simulink model "controller"  (R2024b)
settings: Solver=FixedStepAuto  StartTime=0.0  StopTime=100  FixedStep=1/100  RelTol=1e-3
undefined symbols (not defined in the file or in its folder): MAX_RDB_ENGAGE_SPEED, MAX_TORQUE, MAX_TORQUE_REVERSE, TransmissionState
settings Model: Creator=DAUIN-Win10  LastModifiedBy=aayan
settings SolverCC: AutoInsertRateTranBlk=on
settings OptimizationCC: ReuseModelBlockBuffer=off
settings DebuggingCC: UnconnectedInputMsg=warning  UnconnectedOutputMsg=warning  UnconnectedLineMsg=warning
settings ModelReferenceCC: EnableRefExpFcnMdlSchedulingChecks=on
settings RTWCC: GPUComputeCapability=3.5  DLArmComputeVersion=19.05

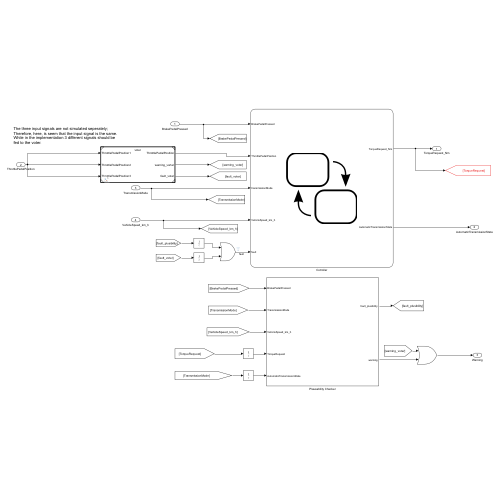
[thumbnail: Simulink's stored preview of the top-level diagram]
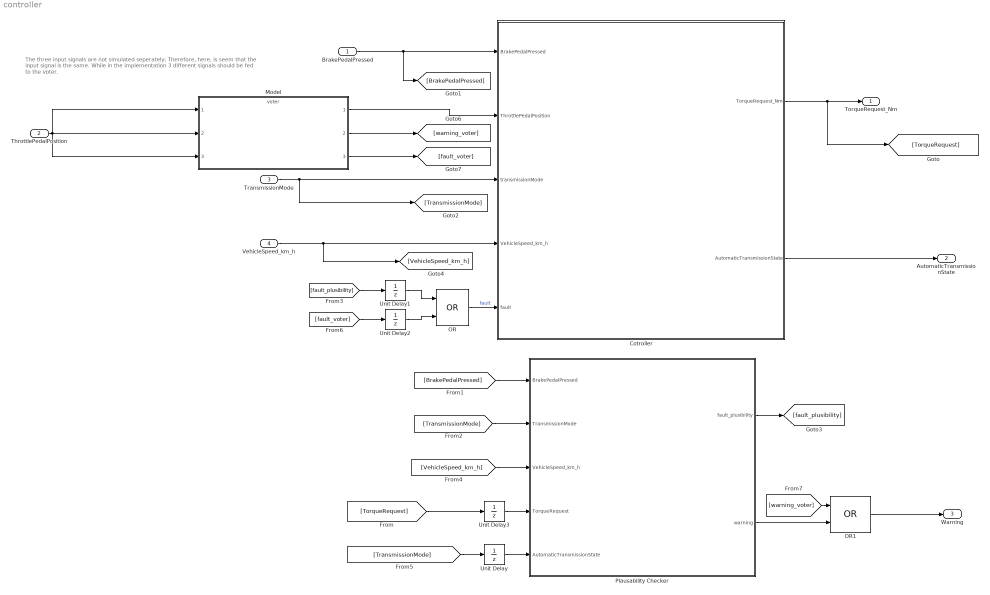
== system controller ==
  note: The three input signals are not simulated seperately;
      | Therefore, here, is seem that the input signal is the same.
      | While in the implementation 3 different signals should be
      | fed to the voter.
  BrakePedalPressed : Inport  OutDataTypeStr=boolean
  ThrottlePedalPosition : Inport  Port=2  OutDataTypeStr=single
  TransmissionMode : Inport  Port=3  OutDataTypeStr=Enum: TransmissionState
  VehicleSpeed_km_h : Inport  Port=4  OutDataTypeStr=single  Unit=km/h
  Cotroller : Stateflow chart  TreatAsAtomicUnit=on
      settings: PortSchema="{\"entries\":[{\"content\":{\"sides\":[{\"content\":{\"connectorIds\":[\"In1\",\"In2\",\"In3\",\"In4\",\"In5\"]},\"type\":\"ConnectorPlacement.EquallySpacedRectSide\",\"uuid\":\"fa3865f3-071a-4523-b56b-dfcb7b7ff1e1\"},{\"content\":{\"connectorIds\":[\"Out2\",\"Out1\"],\"side\":\"RIGHT\"},\"type\":\"ConnectorPlacement.EquallySpacedRectSide\",\"uuid\":\"97edfdd5-6ca1-4319-83ef-4a85a5b2efa4\"},{\"content\":{\"side\":\"TOP\"},\"type\":\"ConnectorPlacement.EquallySpacedRectSide\",\"uuid\":\"bfa350c0-61e1-4051-a5a1-0c01bc7888ec\"}]},\"type\":\"ConnectorPlacement.EquallySpacedConnector\",\"uuid\":\"0069708a-38e0-4c12-a9eb-137e78633e28\"}],\"packageUris\":[\"http://schema.mathworks.com/mf0/Connector/R2020b\"],\"version\":\"1.0\"}"
  Model : ModelReference  ModelNameDialog=voter.slx  SimulationMode=Normal  ModelReferenceVersion=1.25
  OR : Logic  Operator=OR  IconShape=distinctive  AllPortsSameDT=off  OutDataTypeStr=boolean
  OR1 : Logic  Operator=OR  IconShape=distinctive  AllPortsSameDT=off  OutDataTypeStr=boolean
  Plausability Checker : Subsystem
  Unit Delay : UnitDelay  InitialCondition=TransmissionState.Park  SampleTime=-1  HasFrameUpgradeWarning=on
  Unit Delay1 : UnitDelay  SampleTime=-1  HasFrameUpgradeWarning=on
  Unit Delay2 : UnitDelay  SampleTime=-1  HasFrameUpgradeWarning=on
  Unit Delay3 : UnitDelay  SampleTime=-1  HasFrameUpgradeWarning=on
  TorqueRequest_Nm : Outport  OutDataTypeStr=single  Unit=N*m
  AutomaticTransmissionState : Outport  Port=2  OutDataTypeStr=Enum: TransmissionState
  Warning : Outport  Port=3  OutDataTypeStr=boolean
  wires:
  [BrakePedalPressed] -> Plausability Checker/1(BrakePedalPressed)
  [TransmissionMode] -> Plausability Checker/2(TransmissionMode)
  VehicleSpeed_km_h/1 -> [VehicleSpeed_km_h], Cotroller/4(VehicleSpeed_km_h)
  [TorqueRequest] -> Unit Delay3/1
  Plausability Checker/1(fault_plusibility) -> [fault_plusibility]
  [VehicleSpeed_km_h] -> Plausability Checker/3(VehicleSpeed_km_h)
  [TransmissionMode] -> Unit Delay/1
  ThrottlePedalPosition/1 -> Model/3, Model/1, Model/2
  Model/2 -> [warning_voter]
  Model/3 -> [fault_voter]
  OR/1 -> Cotroller/5(fault)  "fault"
  [fault_plusibility] -> Unit Delay1/1
  [fault_voter] -> Unit Delay2/1
  Plausability Checker/2(warning) -> OR1/2
  OR1/1 -> Warning/1
  [warning_voter] -> OR1/1
  BrakePedalPressed/1 -> [BrakePedalPressed], Cotroller/1(BrakePedalPressed)
  TransmissionMode/1 -> [TransmissionMode], Cotroller/3(transmissionMode)
  Model/1 -> Cotroller/2(ThrottlePedalPosition)
  Unit Delay1/1 -> OR/1
  Unit Delay2/1 -> OR/2
  Cotroller/2(TorqueRequest_Nm) -> [TorqueRequest], TorqueRequest_Nm/1
  Cotroller/1(AutomaticTransmissionState) -> AutomaticTransmissionState/1
  Unit Delay/1 -> Plausability Checker/5(AutomaticTransmissionState)
  Unit Delay3/1 -> Plausability Checker/4(TorqueRequest)

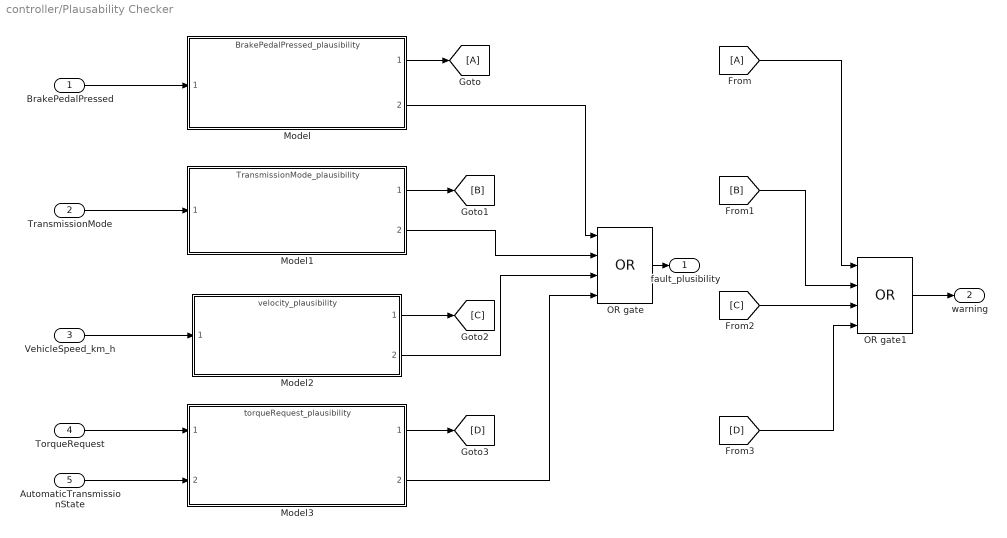
== system controller/Plausability Checker ==
  BrakePedalPressed : Inport
  TransmissionMode : Inport  Port=2  OutDataTypeStr=Enum: TransmissionState
  VehicleSpeed_km_h : Inport  Port=3
  TorqueRequest : Inport  Port=4  OutDataTypeStr=single
  AutomaticTransmissionState : Inport  Port=5  OutDataTypeStr=Enum: TransmissionState
  From : From
  Goto : Goto
  Model : ModelReference  ModelNameDialog=BrakePedalPressed_plausibility.slx  SimulationMode=Normal  ModelReferenceVersion=1.18
  Model1 : ModelReference  ModelNameDialog=TransmissionMode_plausibility.slx  SimulationMode=Normal  ModelReferenceVersion=1.12
  Model2 : ModelReference  ModelNameDialog=velocity_plausibility.slx  SimulationMode=Normal  ModelReferenceVersion=1.13
  Model3 : ModelReference  ModelNameDialog=torqueRequest_plausibility.slx  SimulationMode=Normal  ModelReferenceVersion=1.19
  OR gate : Logic  Operator=OR  Inputs=4  IconShape=distinctive  AllPortsSameDT=off  OutDataTypeStr=boolean
  OR gate1 : Logic  Operator=OR  Inputs=4  IconShape=distinctive  AllPortsSameDT=off  OutDataTypeStr=boolean
  fault_plusibility : Outport  OutDataTypeStr=boolean
  warning : Outport  Port=2
  wires:
  BrakePedalPressed/1 -> Model/1
  Model/1 -> Goto/1
  TransmissionMode/1 -> Model1/1
  Model1/1 -> [B]
  Model/2 -> OR gate/1
  Model1/2 -> OR gate/2
  Model2/2 -> OR gate/3
  AutomaticTransmissionState/1 -> Model3/2
  OR gate1/1 -> warning/1
  Model2/1 -> [C]
  Model3/1 -> [D]
  From/1 -> OR gate1/1
  [B] -> OR gate1/2
  [D] -> OR gate1/4
  [C] -> OR gate1/3
  OR gate/1 -> fault_plusibility/1
  Model3/2 -> OR gate/4
  TorqueRequest/1 -> Model3/1
  VehicleSpeed_km_h/1 -> Model2/1

== stateflow chart controller/Cotroller ==
  settings: updateMethod=DISCRETE  sampleTime=0.01
  state Park
    en:
    AutomaticTransmissionState = TransmissionState.Park;
    du:
    TorqueRequest_Nm = single(0);
  state Neutral
    en:
    AutomaticTransmissionState = TransmissionState.Neutral;
    du:
    TorqueRequest_Nm = single(0);
  state Drive
    en:
    AutomaticTransmissionState = TransmissionState.Drive;
    state ZeroTorque1
      du:
      TorqueRequest_Nm = single(0);
    state Acceleration
      du:
      TorqueRequest_Nm = single(MAX_TORQUE*(ThrottlePedalPosition));
    state StartToMove
      du:
      TorqueRequest_Nm = single(5);
    (default) -> ZeroTorque1
    ZeroTorque1 -> (junction 99) [order 1] : [BrakePedalPressed ~= 1 && VehicleSpeed_km_h  < 5 ]
    (junction 99) -> StartToMove
    (junction 94) -> ZeroTorque1
    StartToMove -> (junction 94) [order 2] : [BrakePedalPressed == 1]
    ZeroTorque1 -> Acceleration [order 2] : [(BrakePedalPressed ~= 1)]
    Acceleration -> ZeroTorque1 : [ (BrakePedalPressed == 1)]
    StartToMove -> Acceleration [order 1] : [ThrottlePedalPosition > 0 && BrakePedalPressed ~= 1]
  state Brake
    en:
    AutomaticTransmissionState = TransmissionState.Brake
    state AccelerationRegion
      du:
      TorqueRequest_Nm = single(MAX_TORQUE*(3/2)*(ThrottlePedalPosition - (1/3)));
    state ZeroTorque
      TorqueRequest_Nm = single(0);
    state DecelerationRegion
      du:
      TorqueRequest_Nm = single(-MAX_TORQUE*(1 - 3*ThrottlePedalPosition));
    (default) -> AccelerationRegion
    Brake.ZeroTorque -> AccelerationRegion : [ThrottlePedalPosition > (1/3)]
    DecelerationRegion -> AccelerationRegion [order 1] : [ (ThrottlePedalPosition >(1/3))]
    AccelerationRegion -> DecelerationRegion : [ ThrottlePedalPosition < (1/3) ]
    (junction 43) -> Brake.ZeroTorque
    DecelerationRegion -> (junction 43) [order 2] : [VehicleSpeed_km_h < MAX_RDB_ENGAGE_SPEED]
  state Reverse
    en:
    AutomaticTransmissionState = TransmissionState.Reverse;
    state Deceleration
      du:
      TorqueRequest_Nm = single(-MAX_TORQUE_REVERSE*(ThrottlePedalPosition));
    state ZeroTorque
      TorqueRequest_Nm = single(0);
    (default) -> Deceleration
    Reverse.ZeroTorque -> Deceleration : [(BrakePedalPressed == 0)]
    Deceleration -> Reverse.ZeroTorque : [(BrakePedalPressed == 1)]
  (default) -> Park
  Neutral -> Drive [order 1] : [(BrakePedalPressed == 1) && (VehicleSpeed_km_h > -5) && ((transmissionMode == TransmissionState.Drive) || (transmissionMode == TransmissionState.Brake)) && fault == 0]
  Park -> Neutral : [(BrakePedalPressed == 1) && (transmissionMode ~= TransmissionState.Park) || fault == 1]
  Drive -> Brake [order 1] : [ThrottlePedalPosition > (1/3) && (transmissionMode == TransmissionState.Brake) && fault == 0]
  Brake -> Drive : [ transmissionMode ~= TransmissionState.Brake || fault == 1]
  Drive -> Neutral [order 2] : [(transmissionMode ~= TransmissionState.Drive) && (transmissionMode ~= TransmissionState.Brake) || fault == 1]
  Neutral -> Park [order 3] : [(BrakePedalPressed == 1) && (abs(VehicleSpeed_km_h) <5) && transmissionMode == TransmissionState.Park && fault == 0]
  Neutral -> Reverse [order 2] : [(BrakePedalPressed == 1) && (VehicleSpeed_km_h < 5) && transmissionMode == 1 && fault == 0]
  Reverse -> Neutral : [transmissionMode ~= TransmissionState.Reverse || fault == 1]
  data: BrakePedalPressed input; ThrottlePedalPosition input; transmissionMode input; VehicleSpeed_km_h input; AutomaticTransmissionState output; TorqueRequest_Nm output; MAX_TORQUE parameter; MAX_TORQUE_REVERSE parameter; MAX_RDB_ENGAGE_SPEED parameter; fault input
